simulink model "Visualizer"  (R2023b)
settings: Solver=FixedStepAuto  StartTime=0.0  StopTime=sim_output(end, 1)  RelTol=1e-12  AbsTol=1e-12
model workspace (MAT data in the model file):
  sim_output = [0 9.54627149192e-15 9.54627149192e-15 4.75923137598e-14 4.75923137598e-14 0.000208333333333 0.00139583333333 0.00164520833333 0.00189458333333 0.00214395833333 0.00289208333333 0.00364020833333 ... (192632 elements, 24079x8)]
libraries: vrlib x1
settings Model: Creator=anigo  LastModifiedBy=anigo
settings OptimizationCC: ReuseModelBlockBuffer=off

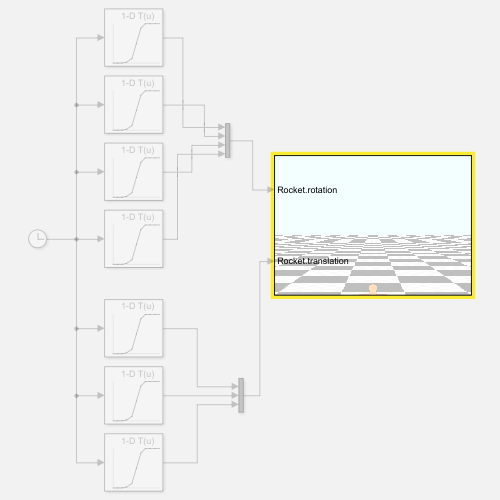
[thumbnail: Simulink's stored preview of the top-level diagram]
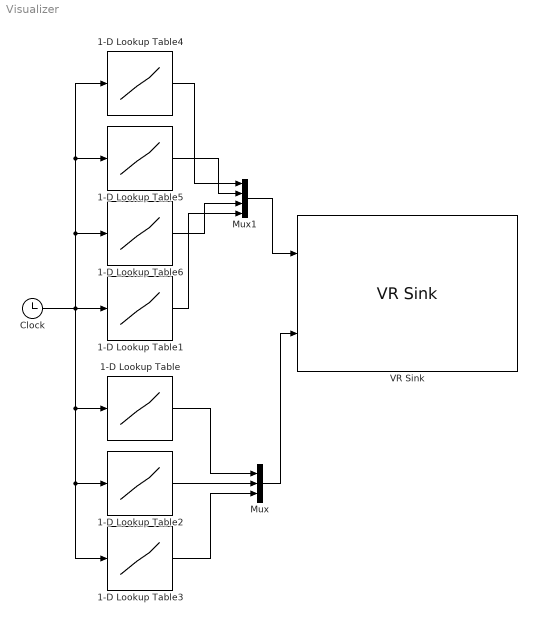
== system Visualizer ==
  1-D Lookup Table : Lookup_n-D  NumberOfTableDimensions=1  BreakpointsForDimension1=sim_output(:, 1)  Table=sim_output(:, 6)  InternalRulePriority=Speed  RndMeth=Simplest
  1-D Lookup Table1 : Lookup_n-D  NumberOfTableDimensions=1  BreakpointsForDimension1=sim_output(:, 1)  Table=sim_output(:, 5)  InternalRulePriority=Speed  RndMeth=Simplest
  1-D Lookup Table2 : Lookup_n-D  NumberOfTableDimensions=1  BreakpointsForDimension1=sim_output(:, 1)  Table=sim_output(:, 7)  InternalRulePriority=Speed  RndMeth=Simplest
  1-D Lookup Table3 : Lookup_n-D  NumberOfTableDimensions=1  BreakpointsForDimension1=sim_output(:, 1)  Table=sim_output(:, 8)  InternalRulePriority=Speed  RndMeth=Simplest
  1-D Lookup Table4 : Lookup_n-D  NumberOfTableDimensions=1  BreakpointsForDimension1=sim_output(:, 1)  Table=sim_output(:, 2)  InternalRulePriority=Speed  RndMeth=Simplest
  1-D Lookup Table5 : Lookup_n-D  NumberOfTableDimensions=1  BreakpointsForDimension1=sim_output(:, 1)  Table=sim_output(:, 3)  InternalRulePriority=Speed  RndMeth=Simplest
  1-D Lookup Table6 : Lookup_n-D  NumberOfTableDimensions=1  BreakpointsForDimension1=sim_output(:, 1)  Table=sim_output(:, 4)  InternalRulePriority=Speed  RndMeth=Simplest
  Clock : Clock
  Mux : Mux  Inputs=3
  Mux1 : Mux
  VR Sink : vrlib/VR Sink  InstantiateOnLoad=on  SampleTime=0.1  ViewEnable=on  RemoteChange=off  RemoteView=off  FieldsWritten=Rocket.rotation.4.1.1.double#Rocket.translation.3.1.1.double  WorldFileName=C:\Users\anigo\OneDrive\Documents\GitHub\Modeling-and-control\assets\world.x3d  AutoView=off  VideoDimensions=[]  AllowVariableSize=off
  wires:
  Clock/1 -> 1-D Lookup Table5/1, 1-D Lookup Table4/1, 1-D Lookup Table6/1, 1-D Lookup Table3/1, 1-D Lookup Table2/1, 1-D Lookup Table/1, 1-D Lookup Table1/1
  1-D Lookup Table2/1 -> Mux/2
  1-D Lookup Table/1 -> Mux/1
  1-D Lookup Table3/1 -> Mux/3
  1-D Lookup Table4/1 -> Mux1/1
  1-D Lookup Table5/1 -> Mux1/2
  1-D Lookup Table6/1 -> Mux1/3
  1-D Lookup Table1/1 -> Mux1/4
  Mux1/1 -> VR Sink/1
  Mux/1 -> VR Sink/2
